simulink library "flatlandHeading_ul"  (R2018a)
settings: Solver=VariableStepAuto  StartTime=0.0  StopTime=10.0  RelTol=1e-3
libraries: dspsigops x1
settings Model: Creator=mcobb  LastModifiedBy=mcobb

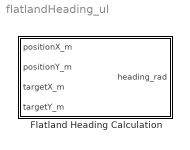
== system flatlandHeading_ul ==
  Flatland Heading Calculation : Subsystem

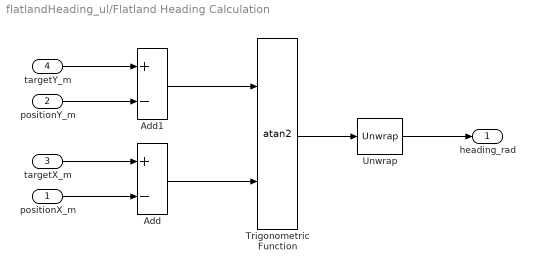
== system flatlandHeading_ul/Flatland Heading Calculation ==
  positionX_m : Inport
  positionY_m : Inport  Port=2
  targetX_m : Inport  Port=3
  targetY_m : Inport  Port=4
  Add : Sum  Inputs=+-
  Add1 : Sum  Inputs=+-
  Trigonometric Function : Trigonometry  Operator=atan2
  Unwrap : dspsigops/Unwrap  tol=pi  InputProcessing=Columns as channels (frame based)  running=off
  heading_rad : Outport
  wires:
  targetX_m/1 -> Add/1
  positionX_m/1 -> Add/2
  targetY_m/1 -> Add1/1
  positionY_m/1 -> Add1/2
  Add1/1 -> Trigonometric Function/1
  Add/1 -> Trigonometric Function/2
  Trigonometric Function/1 -> Unwrap/1
  Unwrap/1 -> heading_rad/1
